simulink model "sensors"  (R2015a)
settings: Solver=ode45  StartTime=0.0  StopTime=10.0  RelTol=1e-3
undefined symbols (not defined in the file or in its folder): accelNoise, accelOffset, dt, gyroMax, gyroNoise, gyroOffset
libraries: simulink x1
settings Model: Creator=johnz  LastModifiedBy=johnz

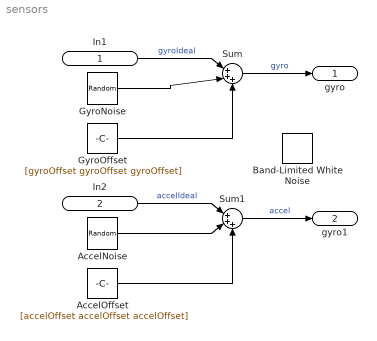
== system sensors ==
  In1 : Inport  OutMin=[-gyroMax]  OutMax=[gyroMax]  OutDataTypeStr=double  PortDimensions=3
  In2 : Inport  Port=2  OutDataTypeStr=double  PortDimensions=3
  AccelNoise : UniformRandomNumber  Minimum=[-accelNoise -accelNoise -accelNoise]  Maximum=[accelNoise accelNoise accelNoise]  Seed=[4 5 6]  SampleTime=dt
  AccelOffset : Constant  Value=[accelOffset accelOffset accelOffset]
  Band-Limited White Noise : simulink/Sources/Band-Limited White Noise  Cov=[0.1]  Ts=0.1  seed=[23341]
  GyroNoise : UniformRandomNumber  Minimum=[-gyroNoise -gyroNoise -gyroNoise]  Maximum=[gyroNoise gyroNoise gyroNoise]  Seed=[1 2 3]  SampleTime=dt
  GyroOffset : Constant  Value=[gyroOffset gyroOffset gyroOffset]
  Sum : Sum  Inputs=|+++
  Sum1 : Sum  Inputs=|+++
  gyro : Outport  OutDataTypeStr=double  PortDimensions=3
  gyro1 : Outport  Port=2  OutDataTypeStr=double  PortDimensions=3
  wires:
  GyroNoise/1 -> Sum/2
  In1/1 -> Sum/1  "gyroIdeal"
  AccelNoise/1 -> Sum1/2
  In2/1 -> Sum1/1  "accelIdeal"
  GyroOffset/1 -> Sum/3
  AccelOffset/1 -> Sum1/3
  Sum/1 -> gyro/1  "gyro"
  Sum1/1 -> gyro1/1  "accel"
